simulink model "OL_SC"  (R2024a)
settings: Solver=FixedStepDiscrete  StartTime=0.0  StopTime=3  FixedStep=Ts  RelTol=RelativeTolerance  EnableMultiTasking=on
undefined symbols (not defined in the file): DenZ, NumZ, Ts
libraries: c2837xDlib x1
settings Model: SimulationMode=external  ExtModeTrigDuration=8  Creator=Fernand  LastModifiedBy=cesar
settings DataIOCC: SaveFormat=StructureWithTime  ReturnWorkspaceOutputs=off  OutputSaveName=data_results  SignalLoggingName=DataResult
settings OptimizationCC: DefaultUnderspecifiedDataType=single  EnhancedBackFolding=on  PassReuseOutputArgsAs=Individual arguments  MaxStackSize=1024  OptimizeBlockOrder=speed  DifferentSizesBufferReuse=on  OptimizationCustomize=off  EfficientTunableParamExpr=on
settings DebuggingCC: ParameterTunabilityLossMsg=error
settings HardwareCC: ProdBitPerChar=16  ProdBitPerInt=16  ProdBitPerPointer=32  ProdBitPerSizeT=32  ProdBitPerPtrDiffT=32  ProdLargestAtomicInteger=Integer  ProdLargestAtomicFloat=None  ProdWordSize=16  ProdLongLongMode=on  ProdHWDeviceType=Texas Instruments->C2000  HardwareBoardFeatureSet=SoCBlockset
settings ModelReferenceCC: ModelReferenceNumInstancesAllowed=Single
settings SFSimCC: MATLABDynamicMemAlloc=off
settings RTWCC: Description=Embedded Coder  SystemTargetFile=ert.tlc  HardwareBoard=TI Delfino F28379D LaunchPad  TemplateMakefile=ert_default_tmf  Toolchain=Texas Instruments Code Composer Studio (C2000)  CodeProfilingSaveOptions=MetricsOnly  GPUComputeCapability=3.5
settings CodeAppCC: ForceParamTrailComments=on  IgnoreCustomStorageClasses=off  OperatorAnnotations=on  SimulinkDataObjDesc=on  SFDataObjDesc=on  InsertBlockDesc=on
settings ERTTargetCC: CodeReplacementLibrary=TI C28x  ExtMode=on  ExtModeTransport=4  ExtModeStaticAlloc=on  ExtModeAutomaticAllocSize=off  ExtModeStaticAllocSize=10000  ExtModeMexFile=ext_xcp  ExtModeMexArgs=1 6 5000000  ExtModeIntrfLevel=Level2 - Open

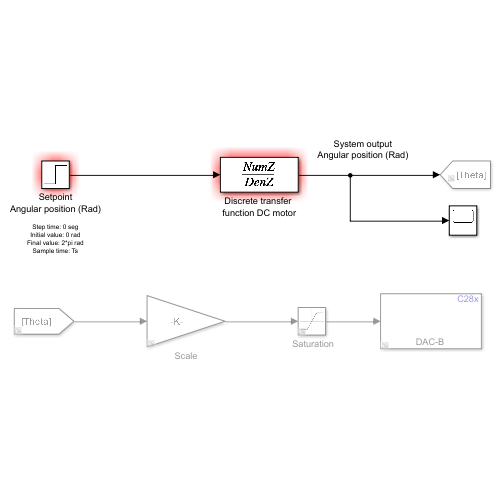
[thumbnail: Simulink's stored preview of the top-level diagram]
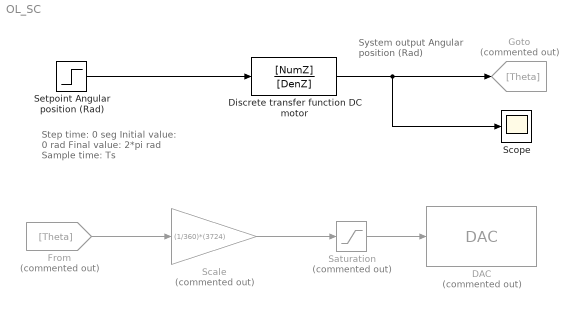
== system OL_SC ==
  note: Step time: 0 seg
      | Initial value: 0 rad
      | Final value: 2*pi rad
      | Sample time: Ts
  note: System output
      | Angular position (Rad)
  " Saturation" : Saturate  Commented=on  UpperLimit=2^12  LowerLimit=0
  DAC : c2837xDlib/DAC  Commented=on  channel=B  saturate=off
  Discrete transfer function DC motor : DiscreteTransferFcn  Numerator=[NumZ]  Denominator=[DenZ]  SampleTime=0.01
  From : From  Commented=on  GotoTag=Theta
  Goto : Goto  Commented=on  GotoTag=Theta
  Scale : Gain  Commented=on  Gain=(1/360)*(3724)  OutDataTypeStr=single
  Scope : Scope
  Setpoint Angular position (Rad) : Step  Time=0  After=2*pi  SampleTime=Ts
  wires:
  Scale/1 -> " Saturation"/1
  From/1 -> Scale/1
  " Saturation"/1 -> DAC/1
  Setpoint Angular position (Rad)/1 -> Discrete transfer function DC motor/1
  Discrete transfer function DC motor/1 -> Scope/1, Goto/1
